simulink model "VOO_old"  (R2020a)
settings: Solver=FixedStepAuto  StartTime=0.0  StopTime=10.0  FixedStep=1e-3  RelTol=1e-3  EnableMultiTasking=on
undefined symbols (not defined in the file): D10, D11, D12, D2, D4, D5, D7, D8, D9, PTA0, PTA2, PTB23, PTB9, PTC3, PTC4, PTD0, PTD2, PTD3
libraries: frdmk64flib x9
settings Model: ExtModeTrigDuration=5  Creator=peter  LastModifiedBy=peter
settings OptimizationCC: EnhancedBackFolding=on  PassReuseOutputArgsAs=Individual arguments  ZeroExternalMemoryAtStartup=off  ZeroInternalMemoryAtStartup=off  MaxStackSize=64  OptimizeBlockOrder=speed  DifferentSizesBufferReuse=on  OptimizationCustomize=off  EfficientTunableParamExpr=on
settings DebuggingCC: ParameterTunabilityLossMsg=error  UnconnectedInputMsg=none  UnconnectedOutputMsg=none  UnconnectedLineMsg=none
settings HardwareCC: ProdBitPerPointer=32  ProdBitPerSizeT=32  ProdBitPerPtrDiffT=32  ProdLargestAtomicInteger=Long  ProdLargestAtomicFloat=Double  ProdWordSize=32  ProdHWDeviceType=ARM Compatible->ARM Cortex
settings ModelReferenceCC: EnableRefExpFcnMdlSchedulingChecks=off
settings SFSimCC: MATLABDynamicMemAlloc=off
settings RTWCC: SystemTargetFile=ert.tlc  HardwareBoard=NXP FRDM-K64F  TemplateMakefile=ert_default_tmf  Toolchain=GNU Tools for ARM Embedded Processors
settings CodeAppCC: ForceParamTrailComments=on  IgnoreCustomStorageClasses=off  OperatorAnnotations=on  SimulinkDataObjDesc=on  SFDataObjDesc=on  InsertBlockDesc=on
settings ERTTargetCC: ExtModeTransport=4  ExtModeMexFile=sendToCommService
settings SettingsController: UseSoCProfilerForTargets=0

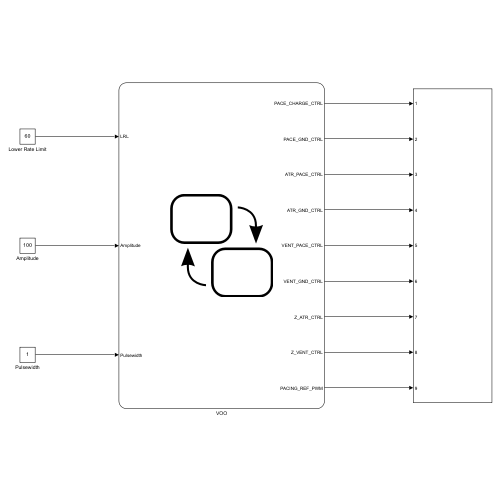
[thumbnail: Simulink's stored preview of the top-level diagram]
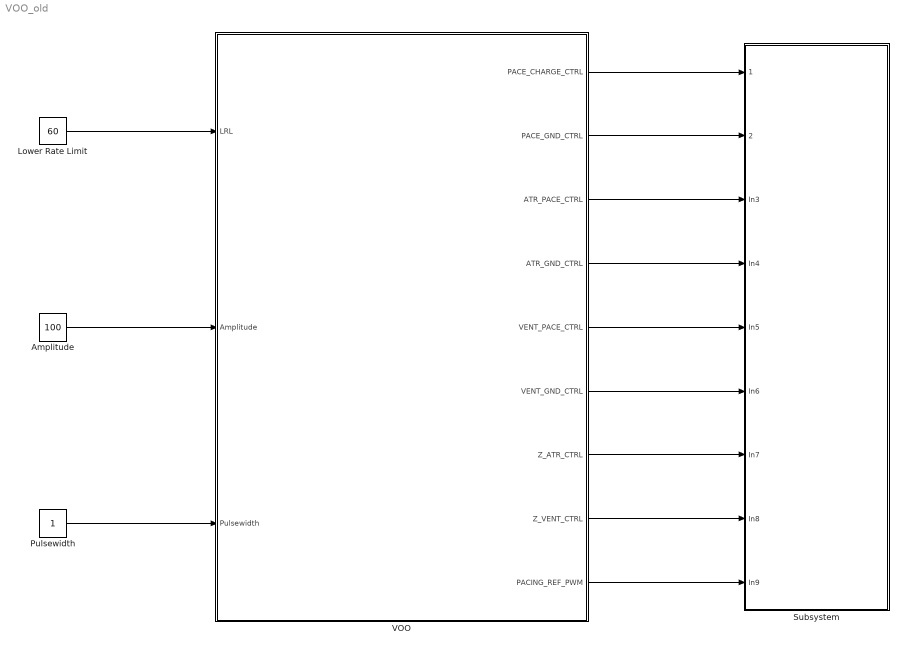
== system VOO_old ==
  Amplitude : Constant  Value=100
  Lower Rate Limit : Constant  Value=60
  Pulsewidth : Constant
  Subsystem : Subsystem
  VOO : Stateflow chart  TreatAsAtomicUnit=on
  wires:
  Lower Rate Limit/1 -> VOO/1(LRL)
  Amplitude/1 -> VOO/2(Amplitude)
  Pulsewidth/1 -> VOO/3(Pulsewidth)
  VOO/1(PACE_CHARGE_CTRL) -> Subsystem/1(1)
  VOO/2(PACE_GND_CTRL) -> Subsystem/2(2)
  VOO/3(ATR_PACE_CTRL) -> Subsystem/3(In3)
  VOO/4(ATR_GND_CTRL) -> Subsystem/4(In4)
  VOO/5(VENT_PACE_CTRL) -> Subsystem/5(In5)
  VOO/6(VENT_GND_CTRL) -> Subsystem/6(In6)
  VOO/7(Z_ATR_CTRL) -> Subsystem/7(In7)
  VOO/8(Z_VENT_CTRL) -> Subsystem/8(In8)
  VOO/9(PACING_REF_PWM) -> Subsystem/9(In9)

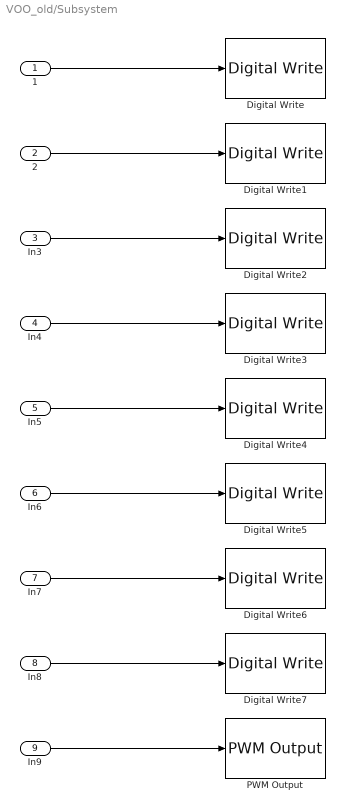
== system VOO_old/Subsystem ==
  1 : Inport
  2 : Inport  Port=2
  In3 : Inport  Port=3
  In4 : Inport  Port=4
  In5 : Inport  Port=5
  In6 : Inport  Port=6
  In7 : Inport  Port=7
  In8 : Inport  Port=8
  In9 : Inport  Port=9
  Digital Write : frdmk64flib/Digital Write  Whichpin=PTB9 (D2)
  Digital Write1 : frdmk64flib/Digital Write  Whichpin=PTD0 (D10)
  Digital Write2 : frdmk64flib/Digital Write  Whichpin=PTA0 (D8)
  Digital Write3 : frdmk64flib/Digital Write  Whichpin=PTD2 (D11)
  Digital Write4 : frdmk64flib/Digital Write  Whichpin=PTC4 (D9)
  Digital Write5 : frdmk64flib/Digital Write  Whichpin=PTD3 (D12)
  Digital Write6 : frdmk64flib/Digital Write  Whichpin=PTB23 (D4)
  Digital Write7 : frdmk64flib/Digital Write  Whichpin=PTC3 (D7)
  PWM Output : frdmk64flib/PWM Output  Whichpin=PTA2 (D5)  InitialFrequency=2000  InitialDutyCycle=100
  wires:
  1/1 -> Digital Write/1
  2/1 -> Digital Write1/1
  In3/1 -> Digital Write2/1
  In4/1 -> Digital Write3/1
  In5/1 -> Digital Write4/1
  In6/1 -> Digital Write5/1
  In7/1 -> Digital Write6/1
  In8/1 -> Digital Write7/1
  In9/1 -> PWM Output/1

== stateflow chart VOO_old/VOO ==
  state Pacing
    entry:
    PACE_CHARGE_CTRL=0;
    PACE_GND_CTRL=1;
    ATR_PACE_CTRL=0;
    ATR_GND_CTRL=0;
    Z_ATR_CTRL=0;
    Z_VENT_CTRL=0;
    VENT_GND_CTRL=0;
    VENT_PACE_CTRL=1;
  state Charging
    entry:
    ATR_PACE_CTRL=0;
    VENT_PACE_CTRL=0;
    PACING_REF_PWM=Amplitude;
    PACE_CHARGE_CTRL=1;
  state Discharging
    entry:
    PACE_GND_CTRL=1;
    VENT_PACE_CTRL=0;
    Z_ATR_CTRL=0;
    Z_VENT_CTRL=0;
    ATR_PACE_CTRL=0;
    ATR_GND_CTRL=0;
    VENT_GND_CTRL=1;
  (default) -> Charging
  Charging -> Pacing : [after(60/LRL,sec)]
  Discharging -> Charging
  Pacing -> Discharging : [after(Pulsewidth,msec)]
  data: LRL input; Amplitude input; Pulsewidth input; PACE_CHARGE_CTRL output; PACE_GND_CTRL output; ATR_PACE_CTRL output; ATR_GND_CTRL output; VENT_PACE_CTRL output; VENT_GND_CTRL output; Z_ATR_CTRL output; Z_VENT_CTRL output; PACING_REF_PWM output
